simulink model "part3"  (R2015a)
settings: Solver=ode3  StartTime=0.0  StopTime=100  FixedStep=0.1  RelTol=1e-8
values from neighbouring files (symbols this model uses):
  K = - place(A, B, [-2 -3 -5 -7])    [create_data.m]
  ue = 0    [create_data.m]
  xe = [0; 0; 0; 0]    [create_data.m]
libraries: simulink x1
settings Model: Creator=vdrouinv  LastModifiedBy=vdrouinv

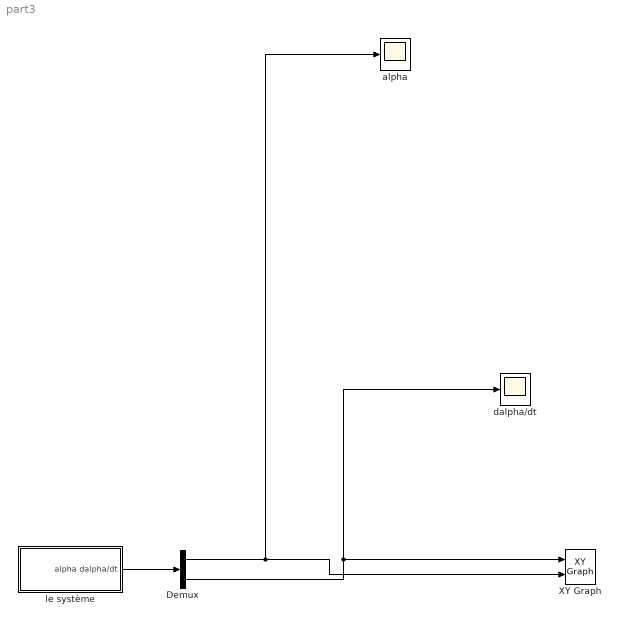
== system part3 ==
  Demux : Demux  Outputs=2
  XY Graph : simulink/Sinks/XY Graph  xmin=-1  xmax=1  ymin=-1  ymax=1  st=-1
  alpha : Scope
  dalpha/dt : Scope
  le système : Subsystem
  wires:
  le système/1(alpha dalpha/dt) -> Demux/1
  Demux/1 -> XY Graph/2, alpha/1
  Demux/2 -> dalpha/dt/1, XY Graph/1

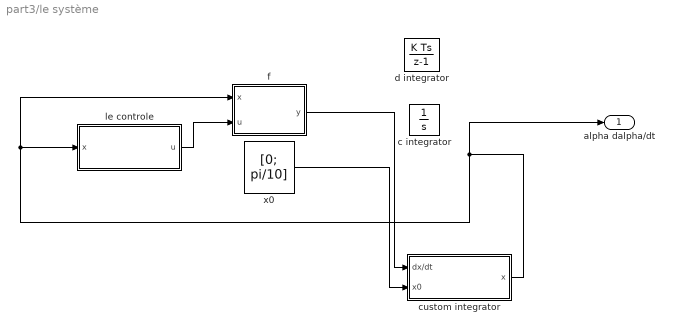
== system part3/le système ==
  c integrator : Integrator  InitialConditionSource=external
  custom integrator : Subsystem  TreatAsAtomicUnit=on
  d integrator : DiscreteIntegrator  InitialConditionSource=external  InitialConditionSetting=State (most efficient)  SampleTime=0.1
  f : MATLAB Function  TreatAsAtomicUnit=on
  le controle : Subsystem  TreatAsAtomicUnit=on
  x0 : Constant  Value=[0; pi/10]
  alpha dalpha/dt : Outport
  wires:
  x0/1 -> custom integrator/2(x0)
  f/1(y) -> custom integrator/1(dx/dt)
  custom integrator/1(x) -> alpha dalpha/dt/1, f/1(x), le controle/1(x)
  le controle/1(u) -> f/2(u)

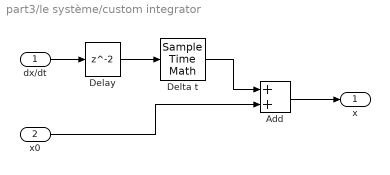
== system part3/le système/custom integrator ==
  dx/dt : Inport
  x0 : Inport  Port=2
  Add : Sum
  Delay : Delay
  Delta t : SampleTimeMath  TsampMathOp=*  weightValue=1
  x : Outport
  wires:
  Delay/1 -> Delta t/1
  Add/1 -> x/1
  x0/1 -> Add/2
  Delta t/1 -> Add/1
  dx/dt/1 -> Delay/1

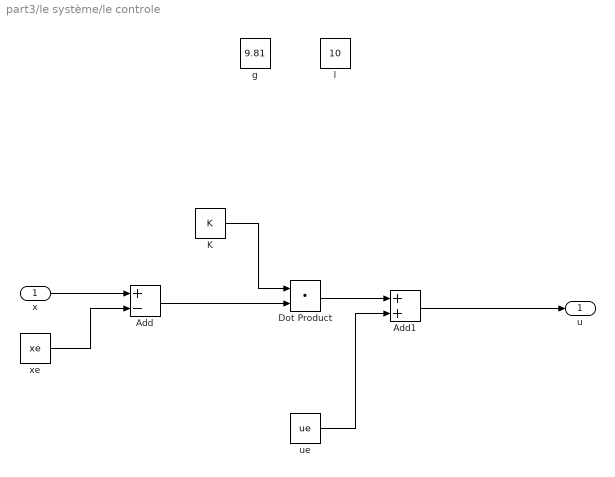
== system part3/le système/le controle ==
  x : Inport
  Add : Sum  Inputs=+-
  Add1 : Sum
  Dot Product : DotProduct  InputSameDT=on  OutDataTypeStr=Inherit: Inherit via internal rule
  K : Constant  Value=K
  g : Constant  Value=9.81
  l : Constant  Value=10
  ue : Constant  Value=ue
  xe : Constant  Value=xe
  u : Outport
  wires:
  x/1 -> Add/1
  xe/1 -> Add/2
  Add/1 -> Dot Product/2
  K/1 -> Dot Product/1
  Dot Product/1 -> Add1/1
  ue/1 -> Add1/2
  Add1/1 -> u/1

== matlab function part3/le système/f ==
  data: x input; u input; y output
function y = f(x, u)

g = 9.81;
l = 10;

y = [x(2); (g/l) * sin(x(1)) - (1/l) * u * cos(x(1))];

end
